simulink model "test_parameter_estimator_simulink"  (R2025b)
settings: Solver=FixedStepDiscrete  StartTime=0.0  StopTime=2.0  FixedStep=0.1  RelTol=1e-3
InitFcn:
  | modelFile = get_param(bdroot, 'FileName'); addpath(fullfile(fileparts(fileparts(modelFile)), 'mex_mdl'));
settings Model: Creator=10120  LastModifiedBy=10120
settings DataIOCC: SignalLogging=off

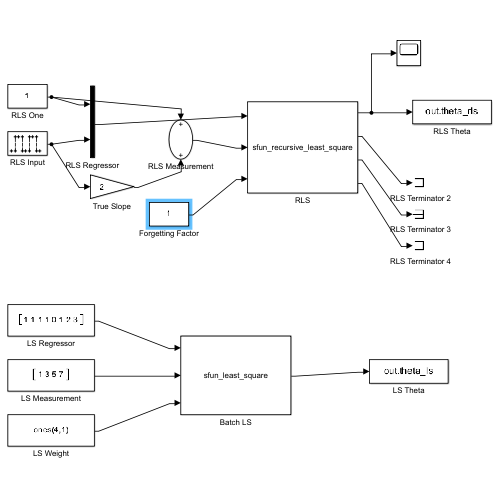
[thumbnail: Simulink's stored preview of the top-level diagram]
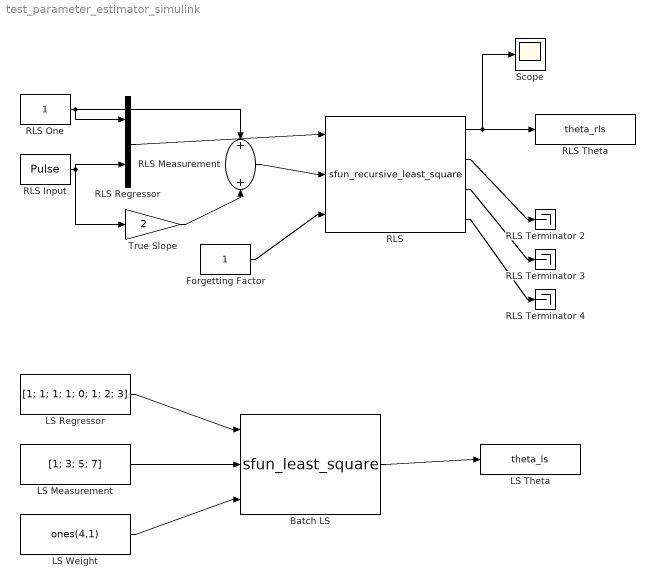
== system test_parameter_estimator_simulink ==
  Batch LS : S-Function  FunctionName=sfun_least_square  SFunctionDeploymentMode=off  EnableBusSupport=off
  Forgetting Factor : Constant
  LS Measurement : Constant  Value=[1; 3; 5; 7]
  LS Regressor : Constant  Value=[1; 1; 1; 1; 0; 1; 2; 3]
  LS Theta : ToWorkspace  VariableName=theta_ls  SaveFormat=Timeseries  SampleTime=-1
  LS Weight : Constant  Value=ones(4,1)
  RLS : S-Function  FunctionName=sfun_recursive_least_square  Parameters=1000  SFunctionDeploymentMode=off  EnableBusSupport=off
  RLS Input : DiscretePulseGenerator  SampleTime=0.1
  RLS Measurement : Sum
  RLS One : Constant
  RLS Regressor : Mux  Inputs=2
  RLS Terminator 2 : Terminator
  RLS Terminator 3 : Terminator
  RLS Terminator 4 : Terminator
  RLS Theta : ToWorkspace  VariableName=theta_rls  SaveFormat=Timeseries  SampleTime=-1
  Scope : Scope
      settings: ActiveDisplayYMinimum=0.87514767431189189  ActiveDisplayYMaximum=2.1246705313029461
  True Slope : Gain  Gain=2
  wires:
  RLS One/1 -> RLS Regressor/1, RLS Measurement/1
  RLS Input/1 -> RLS Regressor/2, True Slope/1
  True Slope/1 -> RLS Measurement/2
  RLS Regressor/1 -> RLS/1
  RLS Measurement/1 -> RLS/2
  Forgetting Factor/1 -> RLS/3
  RLS/1 -> Scope/1, RLS Theta/1
  RLS/2 -> RLS Terminator 2/1
  RLS/3 -> RLS Terminator 3/1
  RLS/4 -> RLS Terminator 4/1
  LS Regressor/1 -> Batch LS/1
  LS Measurement/1 -> Batch LS/2
  LS Weight/1 -> Batch LS/3
  Batch LS/1 -> LS Theta/1
